simulink model "HeliDraft_25_03_2025"  (R2024b)
settings: Solver=VariableStepAuto  StartTime=0.0  StopTime=15  RelTol=1e-3
InitFcn:
  | if exist('MTOW', 'var') == 0
  |     set_param(gcs, 'SimulationCommand', 'stop');
  |     disp('HELICOPTER PARAMETERS ARE NOT DEFINED.');
  | end
values from neighbouring files (symbols this model uses):
  R = D/2    (= 2.01773704722)    [untitled.m]
undefined symbols (not defined in the file or in its folder): AngVel, AngVeltr, BatteryCap, BatteryDischrgRate, Coeffs, Earth, EngPowSL, hRef, Ion, Lfin, Lithium, MTOW, Preq2RPM, RPM2Vreq, VRef, WGS84
libraries: slpidlib x15, simulink x7, fl_lib x7, nesl_utility x6, simulink_extras x3, aerolibatmos2 x2, matrix_library x2, aerolibfltsims x2, aerolibtransform2 x1, shared6dof x1, aerolibconvert2 x1, batteryecm_lib x1
(part 2 of 3)

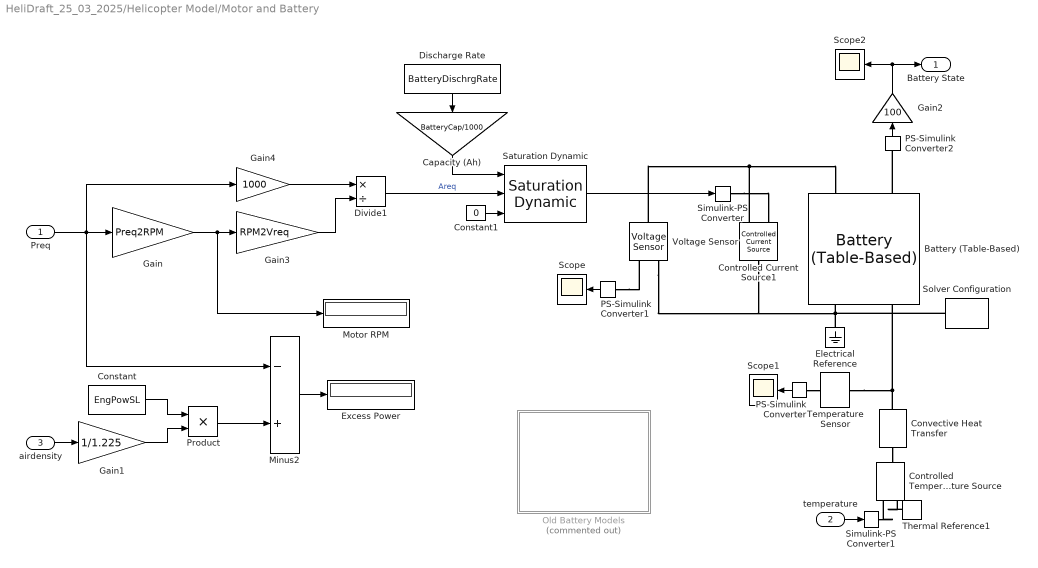
== system HeliDraft_25_03_2025/Helicopter Model/Motor and Battery ==
  Preq : Inport
  temperature : Inport  Port=2
  airdensity : Inport  Port=3
  Battery (Table-Based) : batteryecm_lib/Battery (Table-Based)  PartSpecification="{\"DatasetId\":\"Valence|U27_36XP|simscape.battery.batteryTableBased\",\"DisplayName\":\"Valence:U27_36XP\"}"  SOC_vec=[0 0.01 0.02 0.03 0.04 0.05 0.06 0.07 0.08 0.09 0.1 0.11 0.12 0.13 0.14 0.15 0.16 0.17 0.18 0.19 0.2 0.21 0.22 0.23 0.24 0.25 0.26 0.27 0.28 0.29 0.3 0.31 0.32 0.33 0.34 0.35 0.36 0.37 0.38 0.39 0.4 0.41 0.42 0.43 0.44 0.45 0.46 0.47 0.48 0.49 0.5 0.51 0.52 0.53 0.54 0.55 0.56 0.57 0.58 0.59 0.6 0.61 0.62 0.63 0.64 0.65 0.66 0.67 0.68 0.69 0.7 0.71 0.72 0.73 0.74 0.75 0.76 0.77 0.78 0.79 0.8 0.81 0.82 0.83 0.84 0.85 0.86 0.87 0.88 0.89 0.9 0.91 0.92 0.93 0.94 0.95 0.96 0.97 0.98 0.99 1] % Datasheet derived  T_dependence=simscape.enum.tablebattery.temperature_dependence.no  prm_dir=simscape.enum.tablebattery.prm_dir.noCurrentDirectionality  T_vec=[-10 0 10 20 23 30 40 50] % Datasheet derived degC  V0_mat=[35.84591 35.84591 35.84591 35.84591 35.84591 35.84591 35.84591 35.84591;36.10202 36.10202 36.10202 36.10202 36.10202 36.10202 36.10202 36.10202;36.35814 36.35814 36.35814 36.35814 36.35814 36.35814 36.35814 36.35814;36.61425 36.61425 36.61425 36.61425 36.61425 36.61425 36.61425 36.61425;36.87037 36.87037 36.87037 36.87037 36.87037 36.87037 36.87037 36.87037;37.12649 37.12649 37.12649 37.12649 37.12649 37.12649 37.12649 37.12649;37.3826 37.3826 37.3826 37.3826 37.3826 37.3826 37.3826 37.3826;37.63872 37.63872 37.63872 37.63872 37.63872 37.63872 37.63872 37.63872;37.89483 37.89483 37.89483 37.89483 37.89483 37.89483 37.89483 37.89483;38.09951 38.09951 38.09951 38.09951 38.09951 38.09951 38.09951 38.09951;38.20904 38.20904 38.20904 38.20904 38.20904 38.20904 38.20904 38.20904;38.28916 38.28916 38.28916 38.28916 38.28916 38.28916 38.28916 38.28916;38.37306 38.37306 38.37306 38.37306 38.37306 38.37306 38.37306 38.37306;38.42308 38.42308 38.42308 38.42308 38.42308 38.42308 38.42308 38.42308;38.45482 38.45482 38.45482 38.45482 38.45482 38.45482 38.45482 38.45482;38.47744 38.47744 38.47744 38.47744 38.47744 38.47744 38.47744 38.47744;38.49779 38.49779 38.49779 38.49779 38.49779 38.49779 38.49779 38.49779;38.54815 38.54815 38.54815 38.54815 38.54815 38.54815 38.54815 38.54815;38.5883 38.5883 38.5883 38.5883 38.5883 38.5883 38.5883 38.5883;38.63829 38.63829 38.63829 38.63829 38.63829 38.63829 38.63829 38.63829;38.68732 38.68732 38.68732 38.68732 38.68732 38.68732 38.68732 38.68732;38.72975 38.72975 38.72975 38.72975 38.72975 38.72975 38.72975 38.72975;38.77111 38.77111 38.77111 38.77111 38.77111 38.77111 38.77111 38.77111;38.80795 38.80795 38.80795 38.80795 38.80795 38.80795 38.80795 38.80795;38.83724 38.83724 38.83724 38.83724 38.83724 38.83724 38.83724 38.83724;38.8617 38.8617 38.8617 38.8617 38.8617 38.8617 38.8617 38.8617;38.89023 38.89023 38.89023 38.89023 38.89023 38.89023 38.89023 38.89023;38.9273 38.9273 38.9273 38.9273 38.9273 38.9273 38.9273 38.9273;38.96054 38.96054 38.96054 38.96054 38.96054 38.96054 38.96054 38.96054;38.98786 38.98786 38.98786 38.98786 38.98786 38.98786 38.98786 38.98786;39.01519 39.01519 39.01519 39.01519 39.01519 39.01519 39.01519 39.01519;39.03864 39.03864 39.03864 39.03864 39.03864 39.03864 39.03864 39.03864;39.06385 39.06385 39.06385 39.06385 39.06385 39.06385 39.06385 39.06385;39.08223 39.08223 39.08223 39.08223 39.08223 39.08223 39.08223 39.08223;39.1006 39.1006 39.1006 39.1006 39.1006 39.1006 39.1006 39.1006;39.11898 39.11898 39.11898 39.11898 39.11898 39.11898 39.11898 39.11898;39.13735 39.13735 39.13735 39.13735 39.13735 39.13735 39.13735 39.13735;39.15508 39.15508 39.15508 39.15508 39.15508 39.15508 39.15508 39.15508;39.16412 39.16412 39.16412 39.16412 39.16412 39.16412 39.16412 39.16412;39.17437 39.17437 39.17437 39.17437 39.17437 39.17437 39.17437 39.17437;39.18528 39.18528 39.18528 39.18528 39.18528 39.18528 39.18528 39.18528;39.19619 39.19619 39.19619 39.19619 39.19619 39.19619 39.19619 39.19619;39.20709 39.20709 39.20709 39.20709 39.20709 39.20709 39.20709 39.20709;39.21696 39.21696 39.21696 39.21696 39.21696 39.21696 39.21696 39.21696;39.22232 39.22232 39.22232 39.22232 39.22232 39.22232 39.22232 39.22232;39.22753 39.22753 39.22753 39.22753 39.22753 39.22753 39.22753 39.22753;39.23277 39.23277 39.23277 39.23277 39.23277 39.23277 39.23277 39.23277;39.23672 39.23672 39.23672 39.23672 39.23672 39.23672 39.23672 39.23672;39.23942 39.23942 39.23942 39.23942 39.23942 39.23942 39.23942 39.23942;39.24211 39.24211 39.24211 39.24211 39.24211 39.24211 39.24211 39.24211;39.24481 39.24481 39.24481 39.24481 39.24481 39.24481 39.24481 39.24481;39.24786 39.24786 39.24786 39.24786 39.24786 39.24786 39.24786 39.24786;39.25094 39.25094 39.25094 39.25094 39.25094 39.25094 39.25094 39.25094;39.2539 39.2539 39.2539 39.2539 39.2539 39.2539 39.2539 39.2539;39.25686 39.25686 39.25686 39.25686 39.25686 39.25686 39.25686 39.25686;39.26099 39.26099 39.26099 39.26099 39.26099 39.26099 39.26099 39.26099;39.26708 ...(+3199 chars)] % Datasheet derived V  V0_vec=[62.17 62.61 63.06 63.50 63.95 64.39 64.83 65.28 65.72 66.08 66.27 66.41 66.55 66.64 66.70 66.73 66.77 66.86 66.93 67.01 67.10 67.17 67.24 67.31 67.36 67.40 67.45 67.51 67.57 67.62 67.67 67.71 67.75 67.78 67.82 67.85 67.88 67.91 67.93 67.94 67.96 67.98 67.99 68.02 68.03 68.04 68.04 68.05 68.06 68.07 68.07 68.08 68.08 68.09 68.09 68.09 68.10 68.12 68.13 68.15 68.16 68.19 68.22 68.25 68.28 68.31 68.35 68.39 68.44 68.49 68.54 68.60 68.65 68.69 68.72 68.75 68.77 68.80 68.82 68.84 68.85 68.86 68.87 68.87 68.87 68.86 68.87 68.87 68.89 68.90 68.92 68.92 68.91 68.91 68.91 68.92 68.94 68.95 69.05 69.39 69.91] V  V_range=[50 Inf] % Datasheet derived V  R0_mat=[0.9112 0.73319 0.55116 0.3909 0.47635 0.31145 0.24894 0.23351;0.9112 0.79214 0.50936 0.32708 0.41138 0.21289 0.15029 0.11642;0.9112 0.75838 0.46755 0.26325 0.35007 0.14203 0.09214 0.07324;0.9112 0.72463 0.42575 0.19942 0.29417 0.09634 0.05758 0.04021;0.9112 0.69087 0.38395 0.15149 0.24882 0.06764 0.03364 0.02182;0.9112 0.65711 0.34215 0.11725 0.2142 0.04885 0.01957 0.00983;0.9112 0.62335 0.30035 0.09581 0.18886 0.03484 0.01134 0.00372;0.88245 0.58959 0.25855 0.08105 0.17031 0.02886 0.01013 0.00445;0.85369 0.55583 0.22327 0.07125 0.1569 0.02915 0.01483 0.00976;0.82493 0.52207 0.19506 0.06386 0.14398 0.03152 0.0196 0.01392;0.79618 0.48831 0.16793 0.05824 0.13028 0.031 0.02172 0.01735;0.76742 0.45455 0.14437 0.05231 0.11716 0.03152 0.02306 0.0196;0.73866 0.42079 0.12447 0.04884 0.10632 0.03219 0.02454 0.02192;0.70991 0.38703 0.1096 0.04638 0.09512 0.03151 0.02458 0.0216;0.68115 0.35327 0.09525 0.04318 0.08414 0.02987 0.02387 0.02054;0.65239 0.31952 0.08121 0.03996 0.07347 0.02787 0.02226 0.01912;0.62364 0.27915 0.07388 0.03692 0.06467 0.02578 0.02045 0.01757;0.59488 0.24506 0.06774 0.03508 0.05964 0.02492 0.01984 0.01722;0.56612 0.21466 0.06284 0.03384 0.05477 0.02422 0.01882 0.01646;0.53737 0.18917 0.06009 0.03346 0.05154 0.02391 0.0187 0.0161;0.50861 0.16681 0.05729 0.03301 0.04841 0.02357 0.0188 0.0157;0.47986 0.14646 0.05423 0.03228 0.04625 0.02296 0.01864 0.01586;0.4511 0.13143 0.05231 0.0315 0.04448 0.02305 0.01844 0.01609;0.42234 0.11995 0.05123 0.03055 0.04297 0.02298 0.01851 0.01613;0.39359 0.10903 0.04985 0.03032 0.04112 0.02261 0.01828 0.01587;0.36483 0.09944 0.04828 0.02989 0.03908 0.02204 0.01786 0.01541;0.33607 0.09353 0.04687 0.02963 0.0378 0.02164 0.01762 0.01512;0.30291 0.08834 0.04648 0.02972 0.03771 0.02158 0.01779 0.01527;0.27067 0.08411 0.04619 0.02964 0.03746 0.0219 0.0178 0.01525;0.24264 0.08054 0.04566 0.02987 0.03699 0.02206 0.01758 0.015;0.21621 0.07803 0.04513 0.03012 0.03652 0.02222 0.01736 0.01476;0.19063 0.07544 0.04456 0.03022 0.03598 0.02223 0.01698 0.01435;0.17492 0.07417 0.04451 0.03039 0.03587 0.0223 0.01675 0.01402;0.15924 0.07263 0.04418 0.03029 0.03552 0.0221 0.01669 0.01376;0.14506 0.07109 0.04385 0.03019 0.03517 0.0219 0.01663 0.01361;0.13357 0.06955 0.04352 0.03009 0.03481 0.0217 0.01658 0.01346;0.12461 0.0686 0.04319 0.02998 0.03446 0.0215 0.01652 0.01331;0.11872 0.06771 0.04286 0.02995 0.03417 0.02128 0.01643 0.01313;0.11354 0.06648 0.04251 0.02967 0.03358 0.02084 0.016 0.01261;0.10849 0.0653 0.0422 0.02943 0.03336 0.02078 0.01562 0.01213;0.10559 0.06415 0.04193 0.02923 0.03321 0.02075 0.01526 0.01187;0.10269 0.06364 0.04165 0.02902 0.03305 0.02071 0.01515 0.01197;0.09978 0.06339 0.04137 0.02881 0.0329 0.02068 0.01521 0.01208;0.09733 0.06309 0.04105 0.02856 0.0327 0.0206 0.01523 0.01214;0.09518 0.06261 0.0406 0.02813 0.03227 0.02035 0.01507 0.01203;0.09303 0.06213 0.04031 0.0277 0.03186 0.02009 0.01491 0.01191;0.0912 0.06165 0.04003 0.02736 0.03148 0.01983 0.01474 0.01179;0.08999 0.06112 0.0397 0.02706 0.03105 0.01963 0.01452 0.01161;0.08874 0.06053 0.03932 0.02671 0.03058 0.0194 0.01426 0.01139;0.08749 0.05993 0.03893 0.02636 0.03011 0.01916 0.01399 0.01119;0.08652 0.05934 0.03855 0.02601 0.02964 0.01893 0.01372 0.01104;0.08605 0.05876 0.03818 0.02568 0.02918 0.01872 0.01346 0.01091;0.08557 0.05819 0.03788 0.02534 0.02875 0.0185 0.0132 0.01078;0.0851 0.0576 0.03759 0.025 0.02834 0.01828 0.01294 0.01065;0.08479 0.05702 0.0373 0.02466 0.02792 0.01806 0.01268 0.01051;0.08459 0.05663 0.03706 0.0244 0.02762 0.01789 0.01247 0.01042;0.08446 0.0566 0.0369 0.02423 0.02745 0.01779 0.01233 0.01038;0.08442 0.05667 0.03684 0.02414 0.02737 0.01779 0.01229 0.01018;0.08439 0.05674 0.03677 0.02406 0.02729 0.01777 0.01225 0.00997;0.08436 0.05681 0.0367 0.02397 0.02722 0.01767 0.01221 0.00977;0.08463 0.05687 0.03669 0.02389 0.02715 0.01757 0.01218 0.00956;0.08516 0.0572 0.03698 0.02406 0.0274 0.01773 0.0124 0.00962;0.08586 0.0577 0.03744 0.02442 0.02786 0.01806 0.0128 0.00985;0.08657 0.05819 0.0379 ...(+2382 chars)] % Datasheet derived Ohm  R0_vec=[0.47635 0.41138 0.35007 0.29417 0.24882 0.2142 0.18886 0.17031 0.1569 0.14398 0.13028 0.11716 0.10632 0.09512 0.08414 0.07347 0.06467 0.05964 0.05477 0.05154 0.04841 0.04625 0.04448 0.04297 0.04112 0.03908 0.0378 0.03771 0.03746 0.03699 0.03652 0.03598 0.03587 0.03552 0.03517 0.03481 0.03446 0.03417 0.03358 0.03336 0.03321 0.03305 0.0329 0.0327 0.03227 0.03186 0.03148 0.03105 0.03058 0.03011 0.02964 0.02918 0.02875 0.02834 0.02792 0.02762 0.02745 0.02737 0.02729 0.02722 0.02715 0.0274 0.02786 0.0283 0.02854 0.02877 0.02906 0.02956 0.03013 0.0307 0.03135 0.03204 0.03271 0.03308 0.03307 0.03314 0.03323 0.03332 0.03312 0.03288 0.03264 0.03224 0.03172 0.03113 0.03057 0.03001 0.02945 0.02905 0.02924 0.0293 0.02938 0.02923 0.02879 0.02803 0.02792 0.02793 0.02786 0.02652 0.02587 0.02701 0.00941] ./ 3 Ohm  R0_dis_mat=[.0117, .0085, .009; .011, .0085, .009; .0114, .0087, .0092; .0107, .0082, .0088; .0107, .0083, .0091; .0113, .0085, .0089; .0116, .0085, .0089] % Parameter not set Ohm  R0_dis_vec=[.0085, .0085, .0087, .0082, .0083, .0085, .0085] % Parameter not set Ohm  R0_ch_mat=[.0117, .0085, .009; .011, .0085, .009; .0114, .0087, .0092; .0107, .0082, .0088; .0107, .0083, .0091; .0113, .0085, .0089; .0116, .0085, .0089] % Parameter not set Ohm  R0_ch_vec=[.0085, .0085, .0087, .0082, .0083, .0085, .0085] % Parameter not set Ohm  AH=BatteryCap hr*A  prm_leak=simscape.enum.tablebattery.prm_leak.disabled  Rleak_vec=[8000, 7000, 6000] % Parameter not set Ohm  Rleak=7e3 % Parameter not set Ohm  extrapolation_option=simscape.enum.extrapolation.linear  SOC_port=simscape.enum.tablebattery.enable.yes  prm_dyn=simscape.enum.tablebattery.prm_dyn.off  R1_mat=[.0109, .0029, .0013; .0069, .0024, .0012; .0047, .0026, .0013; .0034, .0016, .001; .0033, .0023, .0014; .0033, .0018, .0011; .0028, .0017, .0011] % Parameter not set Ohm  R1_vec=[.0029, .0024, .0026, .0016, .0023, .0018, .0017] % Parameter not set Ohm  tau1_mat=[20, 36, 39; 31, 45, 39; 109, 105, 61; 36, 29, 26; 59, 77, 67; 40, 33, 29; 25, 39, 33] % Parameter not set s  tau1_vec=[36, 45, 105, 29, 77, 33, 39] % Parameter not set s  R2_mat=[.0109, .0029, .0013; .0069, .0024, .0012; .0047, .0026, .0013; .0034, .0016, .001; .0033, .0023, .0014; .0033, .0018, .0011; .0028, .0017, .0011] % Parameter not set Ohm  R2_vec=[.0029, .0024, .0026, .0016, .0023, .0018, .0017] % Parameter not set Ohm  tau2_mat=[20, 36, 39; 31, 45, 39; 109, 105, 61; 36, 29, 26; 59, 77, 67; 40, 33, 29; 25, 39, 33] % Parameter not set s  tau2_vec=[36, 45, 105, 29, 77, 33, 39] % Parameter not set s  R3_mat=[.0109, .0029, .0013; .0069, .0024, .0012; .0047, .0026, .0013; .0034, .0016, .001; .0033, .0023, .0014; .0033, .0018, .0011; .0028, .0017, .0011] % Parameter not set Ohm  R3_vec=[.0029, .0024, .0026, .0016, .0023, .0018, .0017] % Parameter not set Ohm  tau3_mat=[20, 36, 39; 31, 45, 39; 109, 105, 61; 36, 29, 26; 59, 77, 67; 40, 33, 29; 25, 39, 33] % Parameter not set s  tau3_vec=[36, 45, 105, 29, 77, 33, 39] % Parameter not set s  R4_mat=[.0109, .0029, .0013; .0069, .0024, .0012; .0047, .0026, .0013; .0034, .0016, .001; .0033, .0023, .0014; .0033, .0018, .0011; .0028, .0017, .0011] % Parameter not set Ohm  R4_vec=[.0029, .0024, .0026, .0016, .0023, .0018, .0017] % Parameter not set Ohm  tau4_mat=[20, 36, 39; 31, 45, 39; 109, 105, 61; 36, 29, 26; 59, 77, 67; 40, 33, 29; 25, 39, 33] % Parameter not set s  tau4_vec=[36, 45, 105, 29, 77, 33, 39] % Parameter not set s  R5_mat=[.0109, .0029, .0013; .0069, .0024, .0012; .0047, .0026, .0013; .0034, .0016, .001; .0033, .0023, .0014; .0033, .0018, .0011; .0028, .0017, .0011] % Parameter not set Ohm  R5_vec=[.0029, .0024, .0026, .0016, .0023, .0018, .0017] % Parameter not set Ohm  tau5_mat=[20, 36, 39; 31, 45, 39; 109, 105, 61; 36, 29, 26; 59, 77, 67; 40, 33, 29; 25, 39, 33] % Parameter not set s  tau5_vec=[36, 45, 105, 29, 77, 33, 39] % Parameter not set s  prm_fade=simscape.enum.tablebattery.prm_fade.disabled  N0=100 % Parameter not set  dV0=0 % Parameter not set  dR0=0 % Parameter not set  dAH=0 % Parameter not set  dRleak=0 % Parameter not set  dR1=0 % Parameter not set  dR2=0 % Parameter not set  dR3=0 % Parameter not set  dR4=0 % Parameter not set  dR5=0 % Parameter not set  N0vec=[0 49 97 145 193 241 289 337 385 433 481 529 577 625 673 721 769 817 865 913 961 1009 1057 1105 1153 1201 1249 1297 1345 1393 1441 1489 1537 1585 1633 1681 1729 1777 1825 1873 1921 1969 2017 2065 2113 2161 2209 2257 2305 2353 2401 2449 2497 2545 2593 2641 2689 2737 2785 2833 2881 2929 2977 3025 3073 3121 3169 3217 3265 3313 3361 3409 3457 3505 3553 3601 3649 3697 3745 3793 3841 3889 3937 3985 4033 4081 4129 4177 4225 4273 4321 4369 4417 4465 4513 4561 4609 4657 4705 4753] % Datasheet derived  Tfadevec=[298.15, 323.15] % Parameter not set K  dV0vec=[0 -0.3454 -0.6908 -0.9359 -1.1676 -1.2672 -1.3271 -1.3712 -1.3796 -1.388 -1.3952 -1.402 -1.4086 -1.4146 -1.4207 -1.4251 -1.4284 -1.4315 -1.4266 -1.421 -1.4155 -1.4126 -1.4098 -1.4073 -1.4101 -1.4131 -1.4208 -1.4293 -1.4381 -1.447 -1.458 -1.4708 -1.4792 -1.4819 -1.4846 -1.4851 -1.4846 -1.4841 -1.4836 -1.483 -1.4824 -1.4819 -1.4816 -1.4821 -1.4826 -1.4864 -1.4903 -1.4956 -1.5014 -1.5097 -1.5201 -1.5313 -1.5437 -1.5564 -1.5697 -1.5877 -1.609 -1.6303 -1.6517 -1.6733 -1.6925 -1.7109 -1.7294 -1.7531 -1.7804 -1.8107 -1.8457 -1.8808 -1.9156 -1.9505 -1.9835 -2.0164 -2.048 -2.0852 -2.1232 -2.1613 -2.1969 -2.2314 -2.2586 -2.2847 -2.3081 -2.3315 -2.3541 -2.3775 -2.4018 -2.4263 -2.4508 -2.4714 -2.4903 -2.5029 -2.5135 -2.5281 -2.5444 -2.5606 -2.5769 -2.589 -2.5984 -2.6056 -2.6113 -2.617] % Datasheet derived  dR0vec=[0 0 0 0 0 0 0 0 0 0 0 0 0 0 0 0 0 0 0 0 0 0 0 0 0 0 0 0 0 0 0 0 0 0 0 0 0 0 0 0 0 0 0 0 0 0 0 0 0 0 0 0 0 0 0 0 0 0 0 0 0 0 0 0 0 0 0 0 0 0 0 0 0 0 0 0 0 0 0 0 0 0 0 0 0 0 0 0 0 0 0 0 0 0 0 0 0 0 0 0] % Parameter assumed  dAHvec=[0 -0.472 -0.944 -1.416 -1.889 -2.306 -2.716 -3.125 -3.535 -3.944 -4.342 -4.723 -5.104 -5.485 -5.867 -6.248 -6.629 -6.972 -7.314 -7.656 -7.997 -8.339 -8.681 -9.022 -9.457 -9.923 -10.389 -10.855 -11.321 -11.787 -12.254 -12.72 -13.106 -13.491 -13.876 -14.262 -14.647 -15.032 -15.417 -15.837 -16.264 -16.69 -17.116 -17.542 -17.987 -18.438 -18.889 -19.341 -19.792 -20.243 -20.694 -21.177 -21.71 -22.243 -22.776 -23.309 -23.842 -24.376 -24.909 -25.442 -25.915 -26.366 -26.816 -27.266 -27.717 -28.167 -28.617 -29.068 -29.518 -29.968 -30.419 -30.869 -31.319 -31.858 -32.41 -32.961 -33.512 -34.063 -34.615 -35.166 -35.717 -36.269 -36.802 -37.314 -37.826 -38.339 -38.851 -39.363 -39.875 -40.388 -40.9 -41.603 -42.38 -43.158 -43.935 -44.712 -45.49 -46.267 -47.044 -47.822] % Datasheet derived  dRleakvec=[0, 0, 0, 0] % Parameter not set  dR1vec=[0, 0, 0, 0] % Parameter not set  dR2vec=[0, 0, 0, 0] % Parameter not set  dR3vec=[0, 0, 0, 0] % Parameter not set  dR4vec=[0, 0, 0, 0] % Parameter not set  dR5vec=[0, 0, 0, 0] % Parameter not set  dV0mat=[0, 0; 0, 0; 0, 0; 0, 0] % Parameter not set  dR0mat=[0, 0; 0, 0; 0, 0; 0, 0] % Parameter not set  dAHmat=[0, 0; 0, 0; 0, 0; 0, 0] % Parameter not set  dRleakmat=[0, 0; 0, 0; 0, 0; 0, 0] % Parameter not set  dR1mat=[0, 0; 0, 0; 0, 0; 0, 0] % Parameter not set  dR2mat=[0, 0; 0, 0; 0, 0; 0, 0] % Parameter not set  dR3mat=[0, 0; 0, 0; 0, 0; 0, 0] % Parameter not set  dR4mat=[0, 0; 0, 0; 0, 0; 0, 0] % Parameter not set  dR5mat=[0, 0; 0, 0; 0, 0; 0, 0] % Parameter not set  prm_age_modeling=simscape.enum.tablebattery.prm_age_modeling.equation  storage_dt_age_vec=[0] % Parameter not set d  storage_T_age_vec=[273] % Parameter not set K  prm_age_OCV=simscape.enum.tablebattery.prm_age_OCV.OCV  OCV_age=0.9 % Parameter not set  SOC_age=0.6 % Parameter not set  prm_age_resistance=simscape.enum.tablebattery.prm_age.disabled  OCV_scaling_age_resistance=2.2134e6 % Parameter not set  OCV_offset_age_resistance=1.632e6 % Parameter not set  temp_exp_age_resistance=0.515833569 % Parameter not set V  t_exp_age_resistance=0.75 % Parameter not set  T_age_vec_resistance=[273.15, 298.15, 323.15] % Parameter not set K  dt_age_vec_resistance=[0, 90, 180, 270] % Parameter not set d  dR0_age_vec=[0, 0, 0] % Parameter not set  t_meas_dR0_age=100 % Parameter not set d  dR0_age_mat=[0, 0, 0; 0, 0, 0; 0, 0, 0; 0, 0, 0] % Parameter not set  prm_age_capacity=simscape.enum.tablebattery.prm_age.disabled  OCV_scaling_age_capacity=1.5097e07 % Parameter not set  OCV_offset_age_capacity=8.3625e06 % Parameter not set  temp_exp_age_capacity=0.6011 % Parameter not set V  t_exp_age_capacity=0.75 % Parameter not set  T_age_vec_capacity=[273.15, 298.15, 323.15] % Parameter not set K  dt_age_vec_capacity=[0, 90, 180, 270] % Parameter not set d  dAH_age_vec=[0, 0, 0] % Parameter not set  t_meas_dAH_age=100 % Parameter not set d  dAH_age_mat=[0, 0, 0; 0, 0, 0; 0, 0, 0; 0, 0, 0] % Parameter not set  thermal_port=simscape.enum.thermaleffects.model  temperature=298.15 % Parameter not set K  thermal_mass=16830 % Parameter assumed J/K  i_specify=off  i_priority=None  i=0 A  i_nominal_specify=off  i_nominal_value=1  i_nominal_unit=A  v_specify=off  v_priority=None  v=0 V  v_nominal_specify=off  v_nominal_value=1  v_nominal_unit=V  stateOfCharge_specify=off  stateOfCharge_priority=High  stateOfCharge=1  stateOfCharge_nominal_specify=off  stateOfCharge_nominal_value=1  stateOfCharge_nominal_unit=1  num_cycles_specify=off  num_cycles_priority=High  num_cycles=0  num_cycles_nominal_specify=off  num_cycles_nominal_value=1  num_cycles_nominal_unit=1  cell_temperature_specify=off  cell_temperature_priority=High  cell_temperature=15 degC  cell_temperature_nominal_specify=off  cell_temperature_nominal_value=1  cell_temperature_nominal_unit=K
      settings: AttributesFormatString=Valence:U27_36XP
      settings: LibrarySourceBlock=|
      | batt_lib/Cells/Battery
      | (Table-Based)
  Capacity (Ah) : Gain  Gain=BatteryCap/1000
  Constant : Constant  Value=EngPowSL
  Constant1 : Constant  Value=0
  Controlled Temperature Source : fl_lib/Thermal/Thermal Sources/Controlled Temperature Source
  Controlled Current Source1 : fl_lib/Electrical/Electrical Sources/Controlled Current Source
  Convective Heat Transfer : fl_lib/Thermal/Thermal Elements/Convective Heat Transfer  thermal_type=foundation.enum.constant_variable.constant  area=158850 mm^2  heat_tr_coeff=20 W/(K*m^2)  min_heat_tr_coeff=1e-3 W/(K*m^2)  T_specify=off  T_priority=None  T=0 K  T_nominal_specify=off  T_nominal_value=1  T_nominal_unit=K  Q_specify=off  Q_priority=None  Q=0 W  Q_nominal_specify=off  Q_nominal_value=1  Q_nominal_unit=W
  Discharge Rate : Constant  Value=BatteryDischrgRate
  Divide1 : Product  Inputs=*/
  Electrical Reference : fl_lib/Electrical/Electrical Elements/Electrical Reference
  Excess Power : Display
  Gain : Gain  Gain=Preq2RPM
  Gain1 : Gain  Gain=1/1.225
  Gain2 : Gain  Gain=100
  Gain3 : Gain  Gain=RPM2Vreq
  Gain4 : Gain  Gain=1000
  Minus2 : Sum  Inputs=-+
  Motor RPM : Display
  Old Battery Models : Subsystem  Commented=on
  PS-Simulink Converter : nesl_utility/PS-Simulink Converter  PhysicalDomain=network_engine_domain  SubClassName=ps_output  LeftPortType=input  RightPortType=output  PseudoPeriodic=off  Frequencies=[]  VectorFormat=inherit  Unit=inherit  AffineConversion=off
  PS-Simulink Converter1 : nesl_utility/PS-Simulink Converter  PhysicalDomain=network_engine_domain  SubClassName=ps_output  LeftPortType=input  RightPortType=output  PseudoPeriodic=off  Frequencies=[]  VectorFormat=inherit  Unit=inherit  AffineConversion=off
  PS-Simulink Converter2 : nesl_utility/PS-Simulink Converter  PhysicalDomain=network_engine_domain  SubClassName=ps_output  LeftPortType=input  RightPortType=output  PseudoPeriodic=off  Frequencies=[]  VectorFormat=inherit  Unit=inherit  AffineConversion=off
  Product : Product
  Saturation Dynamic : simulink/Discontinuities/Saturation Dynamic  OutMin=[]  OutMax=[]  OutDataTypeStr=Inherit: Same as second input  OutDataType=fixdt(1, 16)  OutScaling=2^-10  DoSatur=off
  Scope : Scope
  Scope1 : Scope
  Scope2 : Scope
  Simulink-PS Converter : nesl_utility/Simulink-PS Converter  PhysicalDomain=network_engine_domain  SubClassName=ps_input  LeftPortType=input  RightPortType=output  PseudoPeriodic=off  Frequencies=[]  NoiseDistribution=none  NoiseParameters=[]  Unit=1  AffineConversion=off  FilteringAndDerivatives=provide  SimscapeFilterOrder=1  InputFilterTimeConstant=0.001  UdotUserProvided=0
  Simulink-PS Converter1 : nesl_utility/Simulink-PS Converter  PhysicalDomain=network_engine_domain  SubClassName=ps_input  LeftPortType=input  RightPortType=output  PseudoPeriodic=off  Frequencies=[]  NoiseDistribution=none  NoiseParameters=[]  Unit=1  AffineConversion=off  FilteringAndDerivatives=provide  SimscapeFilterOrder=1  InputFilterTimeConstant=0.001  UdotUserProvided=0
  Solver Configuration : nesl_utility/Solver Configuration  PhysicalDomain=network_engine_domain  SubClassName=solver  LeftPortType=input  RightPortType=generic  Tones=[]  Harmonics=[]  SimulateNoise=off  Profile=off  UseLocalSampling=off  EnableSwitchedLinearOptims=on  FrequencyDomain=off  UseCCode=off  RelTol=0.001  AbsTol=0.001  MinStep=1e-09  ToWorkspace=off  RevertToSquareIcSolve=off  NumHomotopyIterations=100  PhasorMode=off  PhasorModeNumHarmonics=1  ConsistencySolver=NEWTON_XTOL_AFTER_FTOL  IndexReductionMethod=DerivativeReplacement  DoDC=off  ResidualTolerance=1e-09  ConsistencyTolSource=GLOBAL  ConsistencyAbsTol=0.001  ConsistencyRelTol=0.001  ConsistencyTolFactor=0.001  UseLocalSolver=off  LocalSolverChoice=NE_BACKWARD_EULER_ADVANCER  ResolveIndetEquations=on  FunctionEvalNumThread=1  LocalSolverSampleTime=0.001  DoFixedCost=off  MaxNonlinIter=3  MaxModeIter=2  ComputeImpulses=off  ImpulseIterations=2  LinearAlgebra=auto  LinearAlgebraNumThread=0  EquationFormulation=NE_TIME_EF  DelaysMemoryBudget=1024  AutomaticFiltering=on  FilteringTimeConstant=0.001  PartitionStorageMethod=AS_NEEDED  PartitionMemoryBudget=1024  PartitionMethod=ROBUST  MultibodyUseLocalSolver=off  MultibodyLocalSolverChoice=ODE1  MultibodyLocalSolverSampleTime=0.001
  Temperature Sensor : fl_lib/Thermal/Thermal Sensors/Temperature Sensor  temperature_measure=foundation.enum.MeasurementReference.absolute
      settings: InternalSimscapePortConfiguration="{\"Bottom\":[],\"Left\":[{\"id\":\"A\",\"label\":\"A\",\"type\":\"foundation.thermal.thermal\"}],\"Right\":[{\"id\":\"T\",\"label\":\"T\",\"type\":\"output\"}],\"Top\":[]}"
  Thermal Reference1 : fl_lib/Thermal/Thermal Elements/Thermal Reference
  Voltage Sensor : fl_lib/Electrical/Electrical Sensors/Voltage Sensor
  Battery State : Outport
  wires:
  Constant/1 -> Product/1
  airdensity/1 -> Gain1/1
  Gain1/1 -> Product/2
  Product/1 -> Minus2/2
  Minus2/1 -> Excess Power/1
  Preq/1 -> Gain/1, Minus2/1, Gain4/1
  Gain4/1 -> Divide1/1
  Gain3/1 -> Divide1/2
  Divide1/1 -> Saturation Dynamic/2  "Areq"
  Gain/1 -> Motor RPM/1, Gain3/1
  Discharge Rate/1 -> Capacity (Ah)/1
  Capacity (Ah)/1 -> Saturation Dynamic/1
  Constant1/1 -> Saturation Dynamic/3
  PS-Simulink Converter1/1 -> Scope/1
  PS-Simulink Converter/1 -> Scope1/1
  Saturation Dynamic/1 -> Simulink-PS Converter/1
  temperature/1 -> Simulink-PS Converter1/1
  PS-Simulink Converter2/1 -> Gain2/1
  Gain2/1 -> Scope2/1, Battery State/1
  connections:
  Voltage Sensor/LConn1 -- Battery (Table-Based)/LConn1 -- Controlled Current Source1/RConn2
  Temperature Sensor/LConn1 -- Convective Heat Transfer/LConn1 -- Battery (Table-Based)/RConn2
  Voltage Sensor/RConn2 -- Controlled Current Source1/LConn1 -- Solver Configuration/RConn1 -- Battery (Table-Based)/RConn1 -- Electrical Reference/LConn1
  Battery (Table-Based)/LConn2 -- PS-Simulink Converter2/LConn1
  Simulink-PS Converter/RConn1 -- Controlled Current Source1/RConn1
  PS-Simulink Converter/LConn1 -- Temperature Sensor/RConn1
  PS-Simulink Converter1/LConn1 -- Voltage Sensor/RConn1
  Thermal Reference1/LConn1 -- Controlled Temperature Source/RConn2
  Simulink-PS Converter1/RConn1 -- Controlled Temperature Source/RConn1
  Convective Heat Transfer/RConn1 -- Controlled Temperature Source/LConn1

== system HeliDraft_25_03_2025/Control/Altitude and Attitude Control/Altitude Controller ==
  PosZRef : Inport
  PosZ : Inport  Port=2
  PID Controller3 : slpidlib/PID Controller  Controller=PID  Form=Parallel  TimeDomain=Continuous-time  UseExternalTs=off  SampleTime=-1  IntegratorMethod=Forward Euler  FilterMethod=Forward Euler  ControllerParametersSource=internal  P=0.09  I=0.02  UseKiTs=off  D=1  UseExternalDerivativeSource=off  N=200  UseFilter=on  TunerSelectOption=Transfer Function Based (PID Tuner App)  InitialConditionSource=internal  InitialConditionForIntegrator=0  InitialConditionForFilter=0  DifferentiatorICPrevScaledInput=0  ExternalReset=none  TrackingMode=off  Kt=10  LimitOutput=on  SatLimitsSource=internal  UpperSaturationLimit=0.2  LowerSaturationLimit=0  LinearizeAsGain=on  AntiWindupMode=back-calculation  Kb=10  LimitIntegrator=off  UpperIntegratorSaturationLimit=inf  LowerIntegratorSaturationLimit=-inf  POutMin=[]  POutMax=[]  IOutMin=[]  IOutMax=[]  DOutMin=[]  DOutMax=[]  NOutMin=[]  NOutMax=[]  SumOutMin=[]  SumOutMax=[]  SaturationOutMin=[]  SaturationOutMax=[]  PParamMin=[]  PParamMax=[]  IParamMin=[]  IParamMax=[]  DParamMin=[]  DParamMax=[]  NParamMin=[]  NParamMax=[]  KbParamMin=[]  KbParamMax=[]  KtParamMin=[]  KtParamMax=[]  KbOutMin=[]  KbOutMax=[]  KtOutMin=[]  KtOutMax=[]  IntegratorOutMin=[]  IntegratorOutMax=[]  FilterOutMin=[]  FilterOutMax=[]  SumI1OutMin=[]  SumI1OutMax=[]  SumI2OutMin=[]  SumI2OutMax=[]  SumI3OutMin=[]  SumI3OutMax=[]  SumI4OutMin=[]  SumI4OutMax=[]  SumDOutMin=[]  SumDOutMax=[]  DifferentiatorOutMin=[]  DifferentiatorOutMax=[]  FilterDiffOutCoefMin=[]  FilterDiffOutCoefMax=[]  ReciprocalOutMin=[]  ReciprocalOutMax=[]  SumDenOutMin=[]  SumDenOutMax=[]  SumNumOutMin=[]  SumNumOutMax=[]  DivideOutMin=[]  DivideOutMax=[]  UdiffTsProdOutMin=[]  UdiffTsProdOutMax=[]  NTsProdOutMin=[]  NTsProdOutMax=[]  UintegralTsProdOutMin=[]  UintegralTsProdOutMax=[]  UngainTsProdOutMin=[]  UngainTsProdOutMax=[]  ClampingZeroOutDataTypeStr=Inherit: Inherit via back propagation  ClampingZeroOutMin=[]  ClampingZeroOutMax=[]  FilterDenConstantOutDataTypeStr=Inherit: Inherit via back propagation  FilterDenConstantOutMin=[]  FilterDenConstantOutMax=[]  PCopyOutDataTypeStr=Inherit: Inherit via back propagation  PCopyOutMin=[]  PCopyOutMax=[]  NCopyOutDataTypeStr=Inherit: Inherit via back propagation  NCopyOutMin=[]  NCopyOutMax=[]  IntegratorContinuousStateAttributes=''  IntegratorStateMustResolveToSignalObject=off  IntegratorRTWStateStorageClass=Auto  FilterContinuousStateAttributes=''  FilterStateMustResolveToSignalObject=off  FilterRTWStateStorageClass=Auto  ParallelPVariant=InternalParameters  IdealPVariant=Disabled  IVariant=InternalParameters  DVariant=InternalParameters  IntegratorVariant=Continuous  SatVariant=Enabled  AWVariant=BackCalculation  PCopyVariant=Disabled  TRVariant=Disabled  FdbkBlocksVariant=Forward  IdealPFdbkVariant=Disabled  SatFdbkVariant=Disabled  DerivativeFilterVariant=ContFilter  NVariant=InternalParameters  NCopyVariant=Disabled  FilterICVariant=InternalICsFilter  IntegratorICVariant=InternalICs  ExternalResetVariant=Disabled  TRSumVariant=Passthrough  SumFdbkVariant=Disabled  SumVariant=Sum_PID  TsampFilterVariant=InternalTs  TsampNgainVariant=Passthrough  TsampIntegralVariant=Disabled_SignalSpec  ExternalSaturationOutDataTypeStr=Inherit: Same as second input  DerivativeSourceVariant=ErrorSignal  PreIntVariant=InternalPreInt
  Scope : Scope
  Sum : Sum  Inputs=|+-
  CollectiveM : Outport  VectorParamsAs1DForOutWhenUnconnected=off
  wires:
  PosZ/1 -> Sum/2
  PosZRef/1 -> Sum/1
  Sum/1 -> PID Controller3/1
  PID Controller3/1 -> Scope/1, CollectiveM/1

== system HeliDraft_25_03_2025/Control/Altitude and Attitude Control/Pitch Controller ==
  thetha : Inport
  q : Inport  Port=2
  thethaRef : Inport  Port=3
  PID Controller : slpidlib/PID Controller  Controller=PID  Form=Parallel  TimeDomain=Continuous-time  UseExternalTs=off  SampleTime=-1  IntegratorMethod=Forward Euler  FilterMethod=Forward Euler  ControllerParametersSource=internal  P=2  I=0.01  UseKiTs=off  D=0  UseExternalDerivativeSource=off  N=50  UseFilter=on  TunerSelectOption=Transfer Function Based (PID Tuner App)  InitialConditionSource=internal  InitialConditionForIntegrator=0  InitialConditionForFilter=0  DifferentiatorICPrevScaledInput=0  ExternalReset=none  TrackingMode=off  Kt=10  LimitOutput=on  SatLimitsSource=internal  UpperSaturationLimit=0.21  LowerSaturationLimit=-0.21  LinearizeAsGain=on  AntiWindupMode=back-calculation  Kb=1  LimitIntegrator=off  UpperIntegratorSaturationLimit=inf  LowerIntegratorSaturationLimit=-inf  POutMin=[]  POutMax=[]  IOutMin=[]  IOutMax=[]  DOutMin=[]  DOutMax=[]  NOutMin=[]  NOutMax=[]  SumOutMin=[]  SumOutMax=[]  SaturationOutMin=[]  SaturationOutMax=[]  PParamMin=[]  PParamMax=[]  IParamMin=[]  IParamMax=[]  DParamMin=[]  DParamMax=[]  NParamMin=[]  NParamMax=[]  KbParamMin=[]  KbParamMax=[]  KtParamMin=[]  KtParamMax=[]  KbOutMin=[]  KbOutMax=[]  KtOutMin=[]  KtOutMax=[]  IntegratorOutMin=[]  IntegratorOutMax=[]  FilterOutMin=[]  FilterOutMax=[]  SumI1OutMin=[]  SumI1OutMax=[]  SumI2OutMin=[]  SumI2OutMax=[]  SumI3OutMin=[]  SumI3OutMax=[]  SumI4OutMin=[]  SumI4OutMax=[]  SumDOutMin=[]  SumDOutMax=[]  DifferentiatorOutMin=[]  DifferentiatorOutMax=[]  FilterDiffOutCoefMin=[]  FilterDiffOutCoefMax=[]  ReciprocalOutMin=[]  ReciprocalOutMax=[]  SumDenOutMin=[]  SumDenOutMax=[]  SumNumOutMin=[]  SumNumOutMax=[]  DivideOutMin=[]  DivideOutMax=[]  UdiffTsProdOutMin=[]  UdiffTsProdOutMax=[]  NTsProdOutMin=[]  NTsProdOutMax=[]  UintegralTsProdOutMin=[]  UintegralTsProdOutMax=[]  UngainTsProdOutMin=[]  UngainTsProdOutMax=[]  ClampingZeroOutDataTypeStr=Inherit: Inherit via back propagation  ClampingZeroOutMin=[]  ClampingZeroOutMax=[]  FilterDenConstantOutDataTypeStr=Inherit: Inherit via back propagation  FilterDenConstantOutMin=[]  FilterDenConstantOutMax=[]  PCopyOutDataTypeStr=Inherit: Inherit via back propagation  PCopyOutMin=[]  PCopyOutMax=[]  NCopyOutDataTypeStr=Inherit: Inherit via back propagation  NCopyOutMin=[]  NCopyOutMax=[]  IntegratorContinuousStateAttributes=''  IntegratorStateMustResolveToSignalObject=off  IntegratorRTWStateStorageClass=Auto  FilterContinuousStateAttributes=''  FilterStateMustResolveToSignalObject=off  FilterRTWStateStorageClass=Auto  ParallelPVariant=InternalParameters  IdealPVariant=Disabled  IVariant=InternalParameters  DVariant=InternalParameters  IntegratorVariant=Continuous  SatVariant=Enabled  AWVariant=BackCalculation  PCopyVariant=Disabled  TRVariant=Disabled  FdbkBlocksVariant=Forward  IdealPFdbkVariant=Disabled  SatFdbkVariant=Disabled  DerivativeFilterVariant=ContFilter  NVariant=InternalParameters  NCopyVariant=Disabled  FilterICVariant=InternalICsFilter  IntegratorICVariant=InternalICs  ExternalResetVariant=Disabled  TRSumVariant=Passthrough  SumFdbkVariant=Disabled  SumVariant=Sum_PID  TsampFilterVariant=InternalTs  TsampNgainVariant=Passthrough  TsampIntegralVariant=Disabled_SignalSpec  ExternalSaturationOutDataTypeStr=Inherit: Same as second input  DerivativeSourceVariant=ErrorSignal  PreIntVariant=InternalPreInt
  PID Controller2 : slpidlib/PID Controller  Controller=PID  Form=Parallel  TimeDomain=Continuous-time  UseExternalTs=off  SampleTime=-1  IntegratorMethod=Forward Euler  FilterMethod=Forward Euler  ControllerParametersSource=internal  P=0.3  I=0.05  UseKiTs=off  D=0.15  UseExternalDerivativeSource=off  N=100  UseFilter=on  TunerSelectOption=Transfer Function Based (PID Tuner App)  InitialConditionSource=internal  InitialConditionForIntegrator=0  InitialConditionForFilter=0  DifferentiatorICPrevScaledInput=0  ExternalReset=none  TrackingMode=off  Kt=10  LimitOutput=on  SatLimitsSource=internal  UpperSaturationLimit=0.35  LowerSaturationLimit=-0.35  LinearizeAsGain=on  AntiWindupMode=back-calculation  Kb=1  LimitIntegrator=off  UpperIntegratorSaturationLimit=inf  LowerIntegratorSaturationLimit=-inf  POutMin=[]  POutMax=[]  IOutMin=[]  IOutMax=[]  DOutMin=[]  DOutMax=[]  NOutMin=[]  NOutMax=[]  SumOutMin=[]  SumOutMax=[]  SaturationOutMin=[]  SaturationOutMax=[]  PParamMin=[]  PParamMax=[]  IParamMin=[]  IParamMax=[]  DParamMin=[]  DParamMax=[]  NParamMin=[]  NParamMax=[]  KbParamMin=[]  KbParamMax=[]  KtParamMin=[]  KtParamMax=[]  KbOutMin=[]  KbOutMax=[]  KtOutMin=[]  KtOutMax=[]  IntegratorOutMin=[]  IntegratorOutMax=[]  FilterOutMin=[]  FilterOutMax=[]  SumI1OutMin=[]  SumI1OutMax=[]  SumI2OutMin=[]  SumI2OutMax=[]  SumI3OutMin=[]  SumI3OutMax=[]  SumI4OutMin=[]  SumI4OutMax=[]  SumDOutMin=[]  SumDOutMax=[]  DifferentiatorOutMin=[]  DifferentiatorOutMax=[]  FilterDiffOutCoefMin=[]  FilterDiffOutCoefMax=[]  ReciprocalOutMin=[]  ReciprocalOutMax=[]  SumDenOutMin=[]  SumDenOutMax=[]  SumNumOutMin=[]  SumNumOutMax=[]  DivideOutMin=[]  DivideOutMax=[]  UdiffTsProdOutMin=[]  UdiffTsProdOutMax=[]  NTsProdOutMin=[]  NTsProdOutMax=[]  UintegralTsProdOutMin=[]  UintegralTsProdOutMax=[]  UngainTsProdOutMin=[]  UngainTsProdOutMax=[]  ClampingZeroOutDataTypeStr=Inherit: Inherit via back propagation  ClampingZeroOutMin=[]  ClampingZeroOutMax=[]  FilterDenConstantOutDataTypeStr=Inherit: Inherit via back propagation  FilterDenConstantOutMin=[]  FilterDenConstantOutMax=[]  PCopyOutDataTypeStr=Inherit: Inherit via back propagation  PCopyOutMin=[]  PCopyOutMax=[]  NCopyOutDataTypeStr=Inherit: Inherit via back propagation  NCopyOutMin=[]  NCopyOutMax=[]  IntegratorContinuousStateAttributes=''  IntegratorStateMustResolveToSignalObject=off  IntegratorRTWStateStorageClass=Auto  FilterContinuousStateAttributes=''  FilterStateMustResolveToSignalObject=off  FilterRTWStateStorageClass=Auto  ParallelPVariant=InternalParameters  IdealPVariant=Disabled  IVariant=InternalParameters  DVariant=InternalParameters  IntegratorVariant=Continuous  SatVariant=Enabled  AWVariant=BackCalculation  PCopyVariant=Disabled  TRVariant=Disabled  FdbkBlocksVariant=Forward  IdealPFdbkVariant=Disabled  SatFdbkVariant=Disabled  DerivativeFilterVariant=ContFilter  NVariant=InternalParameters  NCopyVariant=Disabled  FilterICVariant=InternalICsFilter  IntegratorICVariant=InternalICs  ExternalResetVariant=Disabled  TRSumVariant=Passthrough  SumFdbkVariant=Disabled  SumVariant=Sum_PID  TsampFilterVariant=InternalTs  TsampNgainVariant=Passthrough  TsampIntegralVariant=Disabled_SignalSpec  ExternalSaturationOutDataTypeStr=Inherit: Same as second input  DerivativeSourceVariant=ErrorSignal  PreIntVariant=InternalPreInt
  Sum1 : Sum  Inputs=|+-
  Sum2 : Sum  Inputs=|-+
  cyclicLon : Outport  VectorParamsAs1DForOutWhenUnconnected=off
  wires:
  PID Controller/1 -> cyclicLon/1
  Sum2/1 -> PID Controller/1
  q/1 -> Sum2/2
  Sum1/1 -> PID Controller2/1
  thetha/1 -> Sum1/2
  thethaRef/1 -> Sum1/1
  PID Controller2/1 -> Sum2/1
